simulink model "tp3_practica4"  (R2025b)
settings: Solver=VariableStepAuto  StartTime=0.0  StopTime=0.2  RelTol=1e-3
undefined symbols (not defined in the file or in its folder): dspblkCoreblockFVToolHelper, gcbh

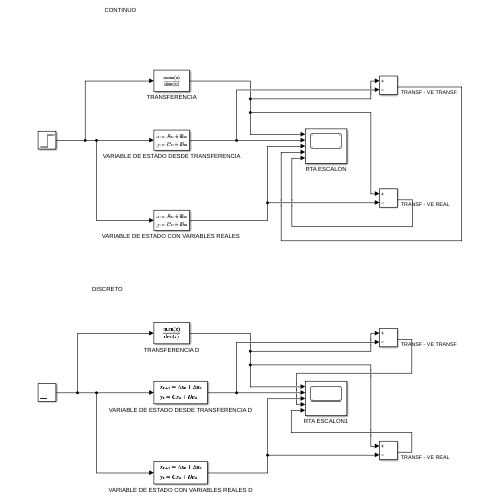
[thumbnail: Simulink's stored preview of the top-level diagram]
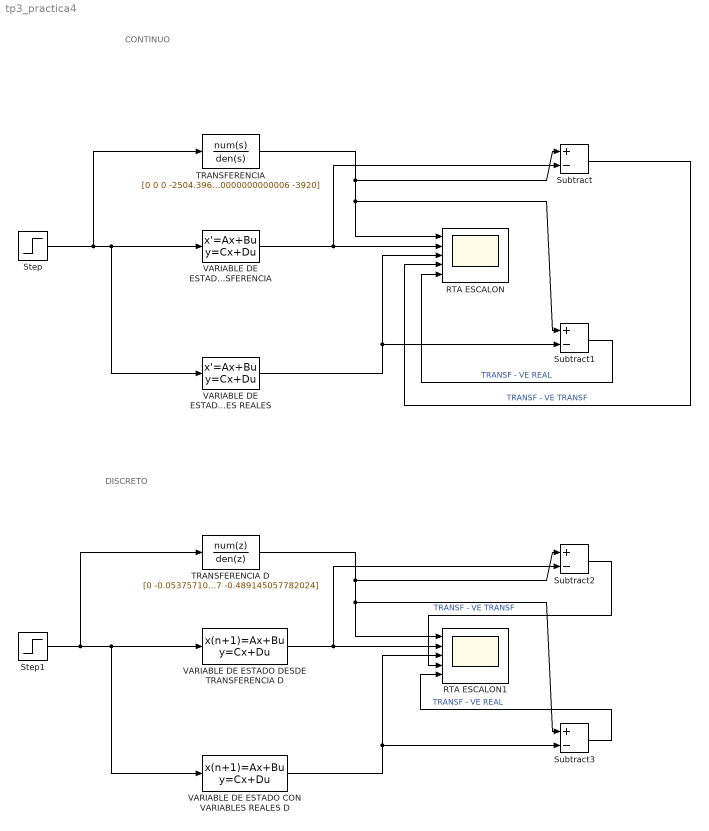
== system tp3_practica4 ==
  note: CONTINUO
  note: DISCRETO
  RTA ESCALON : Scope  NumInputPorts=5
      settings: ActiveDisplayYMinimum=-1.9229062786507711E-13  ActiveDisplayYMaximum=2.5313084961453563E-14  DataLoggingVariableName=ScopeData3
  RTA ESCALON1 : Scope  NumInputPorts=5
      settings: ActiveDisplayYMinimum=-2.4333660510578163E-5  ActiveDisplayYMaximum=0.00021900294459520353
  Step : Step  Time=0  After=0.007826237921249  SampleTime=0
  Step1 : Step  Time=0  After=0.007826237921249  SampleTime=0
  Subtract{,1..3} (4 alike) : Sum  Inputs=+-
  TRANSFERENCIA : TransferFcn  Numerator=[0 0 0 -2504.396134799764]  Denominator=[0.020000000000000 1 -78.400000000000006 -3920]
  TRANSFERENCIA D : DiscreteTransferFcn  LoadFcn=dspblkCoreblockFVToolHelper(gcbh,'load');  Numerator=[0 -0.053757107926140 -0.188445613408456 -0.037448542682443]  Denominator=[1 -3.345989984317583 2.397411576664517 -0.489145057782024]
      settings: CopyFcn=dspblkCoreblockFVToolHelper(gcbh,'copy');  DeleteFcn=dspblkCoreblockFVToolHelper(gcbh,'close');  ModelCloseFcn=dspblkCoreblockFVToolHelper(gcbh,'close');  PreSaveFcn=dspblkCoreblockFVToolHelper(gcbh,'presave');  PostSaveFcn=dspblkCoreblockFVToolHelper(gcbh,'postsave');  CloseFcn=dspblkCoreblockFVToolHelper(gcbh,'close');
  "VARIABLE DE ESTADO CON VARIABLES REALES " : StateSpace  A=[0 1 0;3920 0 -5.008792269599528e+03;0 0 -50]  B=[0;0;25]  C=[1 0 0]  D=0  InitialCondition=0
  VARIABLE DE ESTADO CON VARIABLES REALES D : DiscreteStateSpace  A=[1.428422463267804 0.016291279857016 -0.439904606483240;63.861817039501773 1.428422463267804 -59.604532223658531;0 0 0.489145057782014]  B=[-0.053757190893045;-10.997615162080995;0.255427471108993]  C=[1 0 0]  D=0  SampleTime=0.014301923836314
  VARIABLE DE ESTADO DESDE TRANSFERENCIA : StateSpace  A=[0 1 0;0 0 1;196000 3920 -50]  B=[0;0;-1.252198067399882e+05]  C=[1 0 0]  D=0  InitialCondition=0
  VARIABLE DE ESTADO DESDE TRANSFERENCIA D : DiscreteStateSpace  A=[0 1 0;0 0 1;0.489145057782024 -2.397411576664517 3.345989984317583]  B=[0;0;1]  C=[-0.037448542682443 -0.188445613408456 -0.053757107926140]  D=0  SampleTime=0.014301923836314
  wires:
  "VARIABLE DE ESTADO CON VARIABLES REALES "/1 -> Subtract1/2, RTA ESCALON/3
  VARIABLE DE ESTADO DESDE TRANSFERENCIA/1 -> Subtract/2, RTA ESCALON/2
  Subtract/1 -> RTA ESCALON/4  "TRANSF - VE TRANSF"
  Subtract1/1 -> RTA ESCALON/5  "TRANSF - VE REAL"
  TRANSFERENCIA D/1 -> RTA ESCALON1/1, Subtract3/1, Subtract2/1
  VARIABLE DE ESTADO DESDE TRANSFERENCIA D/1 -> Subtract2/2, RTA ESCALON1/2
  TRANSFERENCIA/1 -> RTA ESCALON/1, Subtract1/1, Subtract/1
  Subtract2/1 -> RTA ESCALON1/4  "TRANSF - VE TRANSF"
  VARIABLE DE ESTADO CON VARIABLES REALES D/1 -> Subtract3/2, RTA ESCALON1/3
  Subtract3/1 -> RTA ESCALON1/5  "TRANSF - VE REAL"
  Step/1 -> TRANSFERENCIA/1, VARIABLE DE ESTADO DESDE TRANSFERENCIA/1, "VARIABLE DE ESTADO CON VARIABLES REALES "/1
  Step1/1 -> TRANSFERENCIA D/1, VARIABLE DE ESTADO CON VARIABLES REALES D/1, VARIABLE DE ESTADO DESDE TRANSFERENCIA D/1
